simulink model "tp2hp_1"  (Simulink 7.7)
settings: Solver=ode45  StartTime=0.0  StopTime=5e-3  MaxStep=1e-5  RelTol=1e-3
values from neighbouring files (symbols this model uses):
  a = zeros(5, nord+1)    [analog_tp1.m]    (also in analog_tp2.m)
  b = fir1(nr-1,0.5)    [adapt_filter1.m]    (also in adapt_filter2.m; analog_tp1.m = zeros(5, nord+1); analog_tp2.m = zeros(5, nord+1))
  Typ = 2    [analog_bp1.m]    (also in analog_bp2.m = 4; analog_bp3.m; analog_tp13.m; analog_tp2.m)
settings Model: Creator=svenhoffmann  LastModifiedBy=josef  ExtModeAutoUpdateStatusClock=off
settings DataIOCC: LimitDataPoints=off  SignalLoggingName=sigsOut
settings DebuggingCC: SaveWithParameterizedLinksMsg=none  SignalResolutionControl=TryResolveAllWithWarning  SolverPrmCheckMsg=none  MultiTaskDSMMsg=warning  MultiTaskCondExecSysMsg=none  StrictBusMsg=None
settings HardwareCC: TargetUnknown=on
settings RTWCC: IncludeERTFirstTime=on

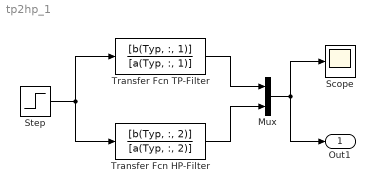
== system tp2hp_1 ==
  Mux : Mux  Inputs=2
  Scope : Scope
  Step : Step  Time=0  SampleTime=0
  Transfer Fcn HP-Filter : TransferFcn  Numerator=[b(Typ, :, 2)]  Denominator=[a(Typ, :, 2)]
  Transfer Fcn TP-Filter : TransferFcn  Numerator=[b(Typ, :, 1)]  Denominator=[a(Typ, :, 1)]
  Out1 : Outport
  wires:
  Step/1 -> Transfer Fcn TP-Filter/1, Transfer Fcn HP-Filter/1
  Transfer Fcn TP-Filter/1 -> Mux/1
  Transfer Fcn HP-Filter/1 -> Mux/2
  Mux/1 -> Scope/1, Out1/1
